simulink model "drone"  (R2017a)
settings: Solver=FixedStepAuto  StartTime=0.0  StopTime=50  FixedStep=0.01  RelTol=1e-3
settings Model: Creator=mrais  LastModifiedBy=mrais

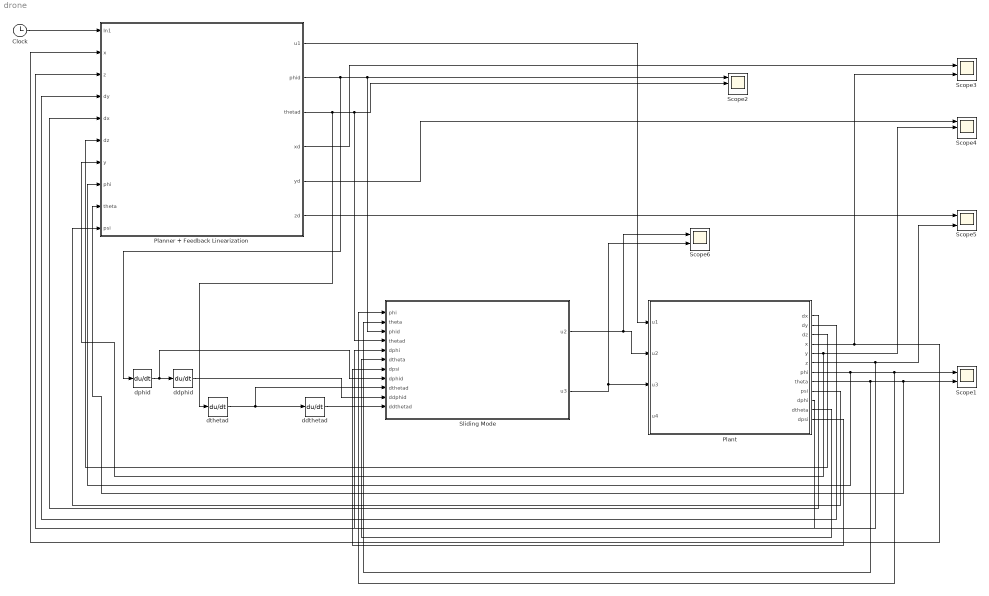
== system drone ==
  Clock : Clock
  Planner + Feedback Linearization : Subsystem
  Plant : Subsystem
  Scope{1,3,5..6} (4 alike) : Scope  NumInputPorts=2
  Scope2 : Scope  NumInputPorts=3
  Scope4 : Scope  NumInputPorts=3
  Sliding Mode : MATLAB Function  TreatAsAtomicUnit=on
  ddphid : Derivative
  ddthetad : Derivative
  dphid : Derivative
  dthetad : Derivative
  wires:
  Plant/7(phi) -> Planner + Feedback Linearization/8(phi), Sliding Mode/1(phi), Scope1/1
  Plant/8(theta) -> Sliding Mode/2(theta), Planner + Feedback Linearization/9(theta), Scope1/2
  Plant/6(z) -> Planner + Feedback Linearization/3(z), Scope5/2
  Clock/1 -> Planner + Feedback Linearization/1(In1)
  Plant/1(dx) -> Planner + Feedback Linearization/5(dx)
  Plant/2(dy) -> Planner + Feedback Linearization/4(dy)
  Plant/3(dz) -> Planner + Feedback Linearization/6(dz)
  Plant/5(y) -> Planner + Feedback Linearization/7(y), Scope4/2
  Plant/12(dpsi) -> Sliding Mode/7(dpsi)
  Planner + Feedback Linearization/3(thetad) -> dthetad/1, Sliding Mode/4(thetad), Scope2/2
  Planner + Feedback Linearization/1(u1) -> Plant/1(u1)
  Plant/10(dphi) -> Sliding Mode/5(dphi)
  Plant/11(dtheta) -> Sliding Mode/6(dtheta)
  Plant/4(x) -> Scope3/2, Planner + Feedback Linearization/2(x)
  Planner + Feedback Linearization/2(phid) -> dphid/1, Sliding Mode/3(phid), Scope2/1
  Planner + Feedback Linearization/4(xd) -> Scope3/1
  Planner + Feedback Linearization/5(yd) -> Scope4/1
  Planner + Feedback Linearization/6(zd) -> Scope5/1
  dphid/1 -> Sliding Mode/8(dphid), ddphid/1
  dthetad/1 -> Sliding Mode/9(dthetad), ddthetad/1
  Plant/9(psi) -> Planner + Feedback Linearization/10(psi)
  ddphid/1 -> Sliding Mode/10(ddphid)
  ddthetad/1 -> Sliding Mode/11(ddthetad)
  Sliding Mode/1(u2) -> Scope6/1, Plant/2(u2)
  Sliding Mode/2(u3) -> Plant/3(u3), Scope6/2

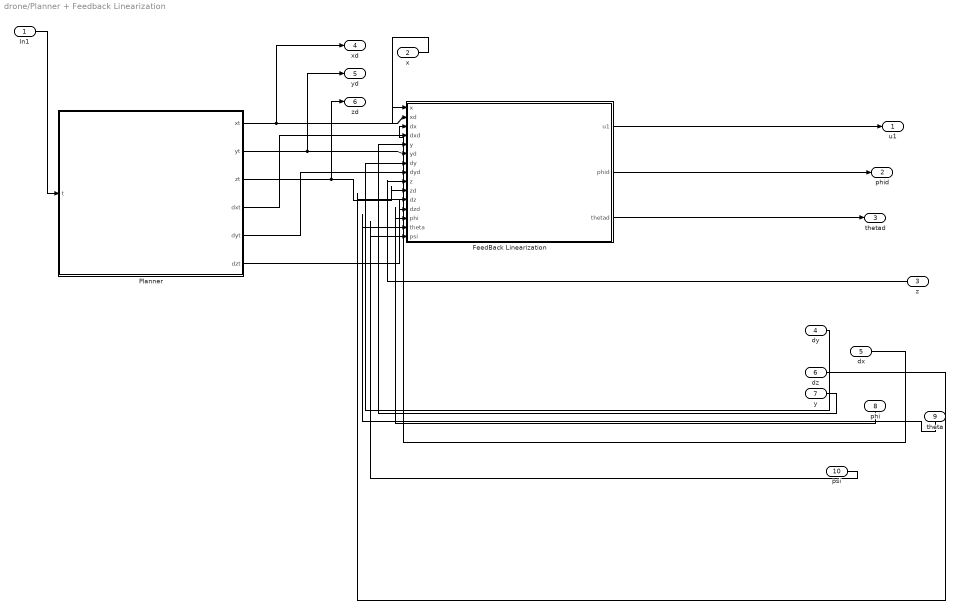
== system drone/Planner + Feedback Linearization ==
  In1 : Inport
  x : Inport  Port=2
  z : Inport  Port=3
  dy : Inport  Port=4
  dx : Inport  Port=5
  dz : Inport  Port=6
  y : Inport  Port=7
  phi : Inport  Port=8
  theta : Inport  Port=9
  psi : Inport  Port=10
  FeedBack Linearization : MATLAB Function  TreatAsAtomicUnit=on
  Planner : MATLAB Function  TreatAsAtomicUnit=on
  u1 : Outport
  phid : Outport  Port=2
  thetad : Outport  Port=3
  xd : Outport  Port=4
  yd : Outport  Port=5
  zd : Outport  Port=6
  wires:
  phi/1 -> FeedBack Linearization/13(phi)
  theta/1 -> FeedBack Linearization/14(theta)
  z/1 -> FeedBack Linearization/9(z)
  x/1 -> FeedBack Linearization/1(x)
  Planner/1(xt) -> xd/1, FeedBack Linearization/2(xd)
  psi/1 -> FeedBack Linearization/15(psi)
  FeedBack Linearization/1(u1) -> u1/1
  Planner/4(dxt) -> FeedBack Linearization/4(dxd)
  FeedBack Linearization/2(phid) -> phid/1
  Planner/2(yt) -> yd/1, FeedBack Linearization/6(yd)
  dy/1 -> FeedBack Linearization/7(dy)
  FeedBack Linearization/3(thetad) -> thetad/1
  y/1 -> FeedBack Linearization/5(y)
  Planner/3(zt) -> zd/1, FeedBack Linearization/10(zd)
  Planner/6(dzt) -> FeedBack Linearization/12(dzd)
  In1/1 -> Planner/1(t)
  Planner/5(dyt) -> FeedBack Linearization/8(dyd)
  dx/1 -> FeedBack Linearization/3(dx)
  dz/1 -> FeedBack Linearization/11(dz)

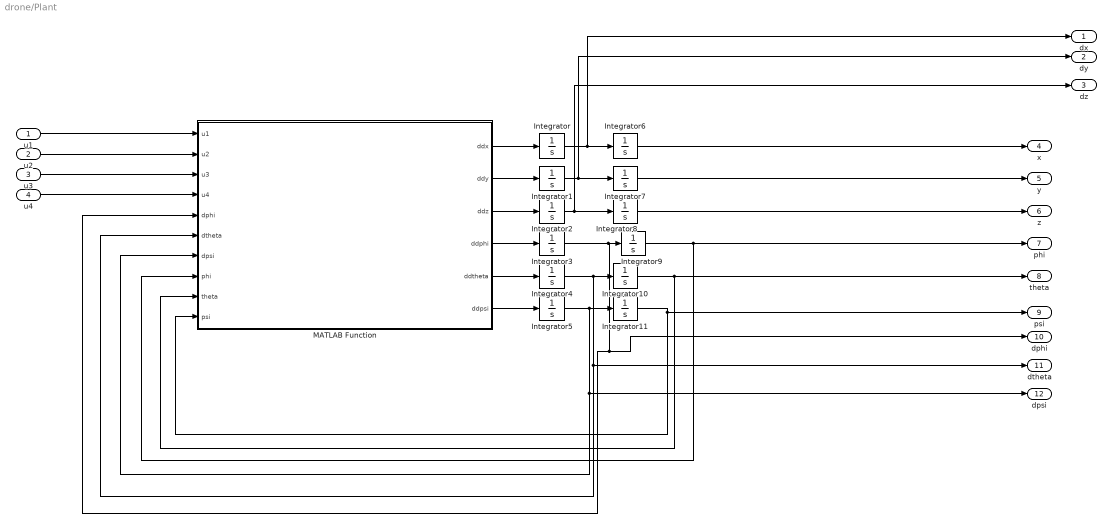
== system drone/Plant ==
  u1 : Inport
  u2 : Inport  Port=2
  u3 : Inport  Port=3
  u4 : Inport  Port=4
  Integrator{,1..11} (12 alike) : Integrator
  MATLAB Function : MATLAB Function  TreatAsAtomicUnit=on
  dx : Outport
  dy : Outport  Port=2
  dz : Outport  Port=3
  x : Outport  Port=4
  y : Outport  Port=5
  z : Outport  Port=6
  phi : Outport  Port=7
  theta : Outport  Port=8
  psi : Outport  Port=9
  dphi : Outport  Port=10
  dtheta : Outport  Port=11
  dpsi : Outport  Port=12
  wires:
  Integrator4/1 -> Integrator10/1, MATLAB Function/6(dtheta), dtheta/1
  MATLAB Function/5(ddtheta) -> Integrator4/1
  Integrator11/1 -> psi/1, MATLAB Function/10(psi)
  Integrator5/1 -> Integrator11/1, dpsi/1, MATLAB Function/7(dpsi)
  Integrator8/1 -> z/1
  u4/1 -> MATLAB Function/4(u4)
  Integrator1/1 -> dy/1, Integrator7/1
  MATLAB Function/1(ddx) -> Integrator/1
  MATLAB Function/4(ddphi) -> Integrator3/1
  u1/1 -> MATLAB Function/1(u1)
  u3/1 -> MATLAB Function/3(u3)
  MATLAB Function/2(ddy) -> Integrator1/1
  MATLAB Function/3(ddz) -> Integrator2/1
  Integrator7/1 -> y/1
  Integrator3/1 -> MATLAB Function/5(dphi), dphi/1, Integrator9/1
  MATLAB Function/6(ddpsi) -> Integrator5/1
  Integrator9/1 -> phi/1, MATLAB Function/8(phi)
  Integrator10/1 -> theta/1, MATLAB Function/9(theta)
  Integrator6/1 -> x/1
  Integrator/1 -> dx/1, Integrator6/1
  Integrator2/1 -> dz/1, Integrator8/1
  u2/1 -> MATLAB Function/2(u2)

== matlab function drone/Sliding Mode ==
  data: phi input; theta input; phid input; thetad input; dphi input; u2 output; dtheta input; dpsi input; dphid input; dthetad input; ddphid input; ddthetad input; u3 output
function [u2, u3] = fcn(phi, theta, phid, thetad, dphi, dtheta, dpsi, dphid, dthetad, ddphid, ddthetad)

constant = initial_constants();
lambda = 10;
l = 1; Jr = constant{6};
Ix = constant{1}; Iy = constant{2}; Iz = constant{3};
Omega = 5000;

ku2 = 10;
ku3 = 10;
su2 = (dphid - dphi) + lambda*(phid - phi);
su3 = (dthetad - dtheta) + lambda*(thetad - theta);

delta = 0.1;
u2 = (lambda*(dphid - dphi) + ddphid - dtheta*dpsi*((Iy-Iz)/Ix) + Jr*dtheta*Omega/Ix)*Ix/l + ku2*(su2/(abs(su2 + delta)));
u3 = (lambda*(dthetad - dtheta) + ddthetad - dphi*dpsi*((Iz-Ix)/Iy) - Jr*dtheta*Omega/Iy)*Iy/l + ku3*(su3/(abs(su3 + delta)));

== matlab function drone/Plant/MATLAB Function ==
  data: ddx output; ddy output; u1 input; u2 input; u3 input; u4 input; ddz output; ddphi output; ddtheta output; ddpsi output; dphi input; dtheta input; dpsi input; phi input; theta input; psi input
function [ddx, ddy, ddz, ddphi, ddtheta, ddpsi] = fcn(u1, u2, u3, u4, dphi, dtheta, dpsi, phi, theta, psi)

constant = initial_constants();
Ix = constant{1}; Iy = constant{2}; Iz = constant{3}; 
m = constant{4};
g = constant{5};
Jr = constant{6};

Omega = 5000;
l = 1; 

ddx = (cos(phi)*sin(theta)*cos(psi) + sin(phi)*sin(psi))*u1/m;
ddy = (cos(phi)*sin(theta)*sin(psi) - sin(phi)*cos(psi))*u1/m;
ddz = -g + cos(phi)*cos(theta)*u1/m;

ddphi = dphi*dpsi*((Iy - Iz)/Ix) - Jr*dtheta*Omega/Ix + l*u2/Ix;
ddtheta = dphi*dpsi*((Iz - Ix)/Iy) + Jr*dtheta*Omega/Iy + l*u3/Iy;
ddpsi = dtheta*dphi*((Ix - Iy)/Iz) + u4/Iz;

== matlab function drone/Planner + Feedback Linearization/Planner ==
  data: xt output; yt output; t input; zt output; dxt output; dyt output; dzt output
function [xt,yt, zt, dxt, dyt, dzt] = fcn(t)
R=10;
zt = R*sin(t/2);
dzt = R*cos(t/2);
xt = R*sin(t/2);
dxt = R*cos(t/2);
yt = 0;
dyt = 0;

end

== matlab function drone/Planner + Feedback Linearization/FeedBack Linearization ==
  data: x input; xd input; dx input; dxd input; y input; yd input; dy input; dyd input; z input; u1 output; zd input; dz input; dzd input; phi input; theta input; phid output; thetad output; psi input
function [u1, phid, thetad] = fcn(x, xd, dx, dxd, y, yd, dy, dyd, z, zd, dz, dzd, phi, theta, psi)
constant = initial_constants();
g = constant{5};
m = constant{4};

k1x = 40; k2x = 40;
k1y = 8; k2y = 16;
k1z = 8; k2z = 16;

vx = k1x*(xd - x) + k2x*(dxd - dx);
vy = k1y*(yd - y) + k2y*(dyd - dy);
vz = k1z*(zd - z) + k2z*(dzd - dz);

a = vx /(vz + g); 
b = vy /(vz + g); 
c = cos(psi);
d = sin(psi);

u1 = (vz + g)*m/(cos(phi)*cos(theta));
thetad = atan(a*c+b*d);

if abs(psi) < pi/4 || abs(psi) > 3*pi/4
    phid = atan( (cos(theta)*(tan(theta)*d - b))/c);
else
    phid = atan( (cos(theta)*(a - tan(theta)*c))/d);
end


end
